simulink library "lib_DCDC"  (R2017a)
settings: Solver=VariableStepAuto  StartTime=0.0  StopTime=10.0  RelTol=1e-3
undefined symbols (not defined in the file): dcdc
settings Model: Creator=Di Russo  LastModifiedBy=Vraj M

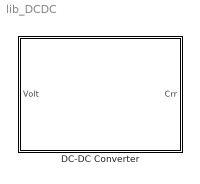
== system lib_DCDC ==
  DC-DC Converter : Subsystem
      mask Display:
      | image('Images/DCDC.PNG')
      | color('red');
      | port_label('Input',1,'Volt')
      | port_label('Output',1,'Crr')

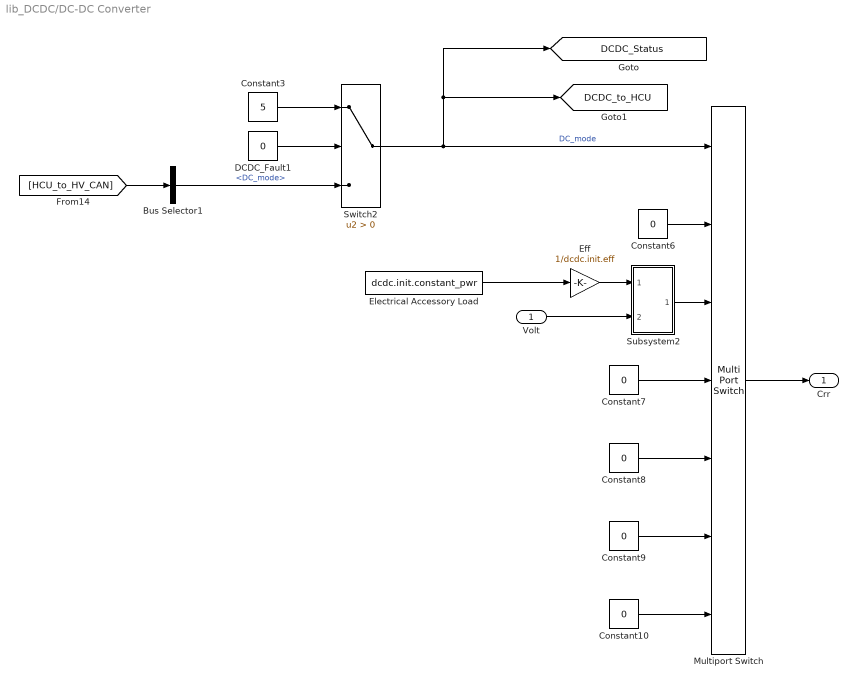
== system lib_DCDC/DC-DC Converter ==
  Volt : Inport
  Bus Selector1 : BusSelector  OutputSignals=DCDC.DC_mode
  Constant{6..10} (5 alike) : Constant  Value=0
  Constant3 : Constant  Value=5
  DCDC_Fault1 : Constant  Value=0
  Eff : Gain  Gain=1/dcdc.init.eff
  Electrical Accessory Load : Constant  Value=dcdc.init.constant_pwr
  Multiport Switch : MultiPortSwitch  DataPortOrder=Zero-based contiguous  Inputs=6  zeroidx=on
  Subsystem2 : Subsystem
      mask Display: disp('divider')
  Switch2 : Switch  Criteria=u2 > Threshold
  Crr : Outport
  tag scope: DCDC_Status=global, DCDC_to_HCU=global
  wires:
  Constant10/1 -> Multiport Switch/7
  Constant9/1 -> Multiport Switch/6
  Constant8/1 -> Multiport Switch/5
  Constant7/1 -> Multiport Switch/4
  Eff/1 -> Subsystem2/1(In1)
  Volt/1 -> Subsystem2/2(In2)
  Subsystem2/1(Out1) -> Multiport Switch/3
  Electrical Accessory Load/1 -> Eff/1
  Constant6/1 -> Multiport Switch/2
  Multiport Switch/1 -> Crr/1
  Constant3/1 -> Switch2/1
  Bus Selector1/1 -> Switch2/3  "<DC_mode>"
  [HCU_to_HV_CAN] -> Bus Selector1/1
  Switch2/1 -> Multiport Switch/1, [DCDC_to_HCU], [DCDC_Status]  "DC_mode"
  DCDC_Fault1/1 -> Switch2/2

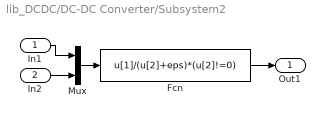
== system lib_DCDC/DC-DC Converter/Subsystem2 ==
  In1 : Inport
  In2 : Inport  Port=2
  Fcn : Fcn  Expr=u[1]/(u[2]+eps)*(u[2]!=0)
  Mux : Mux  Inputs=2
  Out1 : Outport
  wires:
  Mux/1 -> Fcn/1
  In1/1 -> Mux/1
  Fcn/1 -> Out1/1
  In2/1 -> Mux/2
